simulink model "dynamical_model"  (R2023b)
settings: Solver=VariableStepAuto  StartTime=0.0  StopTime=10.0  RelTol=1e-3
values from neighbouring files (symbols this model uses):
  A = double(subs(A,[Lr lp Jr_ex mp Jp g Ke Kc Ra Br Bp],[Lr_ lp_ Jr_ex_ mp_ Jp_ g_ Ke_ Kc_ Ra_ Br_ Bp_]))    [linearized_mechanical_model.m]
  alpha_0 = 0    [DC_motor_and_Rod.m]    (also in linearized_mechanical_model.m)
  B = double(subs(B,[Lr lp Jr_ex mp Jp g Ke Kc Ra Br Bp],[Lr_ lp_ Jr_ex_ mp_ Jp_ g_ Ke_ Kc_ Ra_ Br_ Bp_]))    [linearized_mechanical_model.m]
  Bp_ = 1.25e-5    (= 1.25e-05)    [DC_motor_and_Rod.m]    (also in linearized_mechanical_model.m = 0)
  Br_ = 1.25e-5    (= 1.25e-05)    [DC_motor_and_Rod.m]    (also in linearized_mechanical_model.m = 0)
  C = [1,0,0,0 ... (first row only)    [linearized_mechanical_model.m]
  D = [0 ... (first row only)    [linearized_mechanical_model.m]
  g_ = 9.81    [DC_motor_and_Rod.m]    (also in linearized_mechanical_model.m)
  Jp_ = (1/12)*mp_*(3*rp^2 + Lp^2)    (= 3.3718538025e-05)    [DC_motor_and_Rod.m]    (also in linearized_mechanical_model.m = 2.44e-05)
  Jr_ex_ = 9.5e-5 + Jm    (= 9.96e-05)    [DC_motor_and_Rod.m]    (also in linearized_mechanical_model.m = 9.5e-05)
  Kc_ = 0.042    [DC_motor_and_Rod.m]    (also in linearized_mechanical_model.m)
  Ke_ = 0.042    [DC_motor_and_Rod.m]    (also in linearized_mechanical_model.m)
  lp_ = 0.95*Lp/2    (= 0.061275)    [DC_motor_and_Rod.m]    (also in linearized_mechanical_model.m = 0.0645)
  Lr_ = 0.09    [DC_motor_and_Rod.m]    (also in linearized_mechanical_model.m = 0.085)
  mp_ = 0.02421    [DC_motor_and_Rod.m]    (also in linearized_mechanical_model.m = 0.024)
  Ra_ = 8.4    [DC_motor_and_Rod.m]    (also in linearized_mechanical_model.m)
  theta_0 = 0    [DC_motor_and_Rod.m]    (also in linearized_mechanical_model.m)
  Va_0 = 0    [linearized_mechanical_model.m]
settings Model: Creator=renzo  LastModifiedBy=renzo

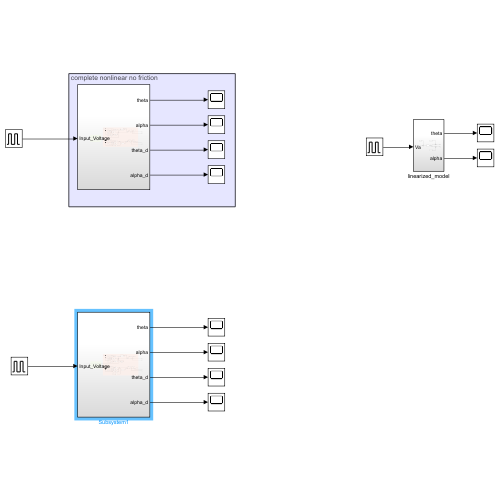
[thumbnail: Simulink's stored preview of the top-level diagram]
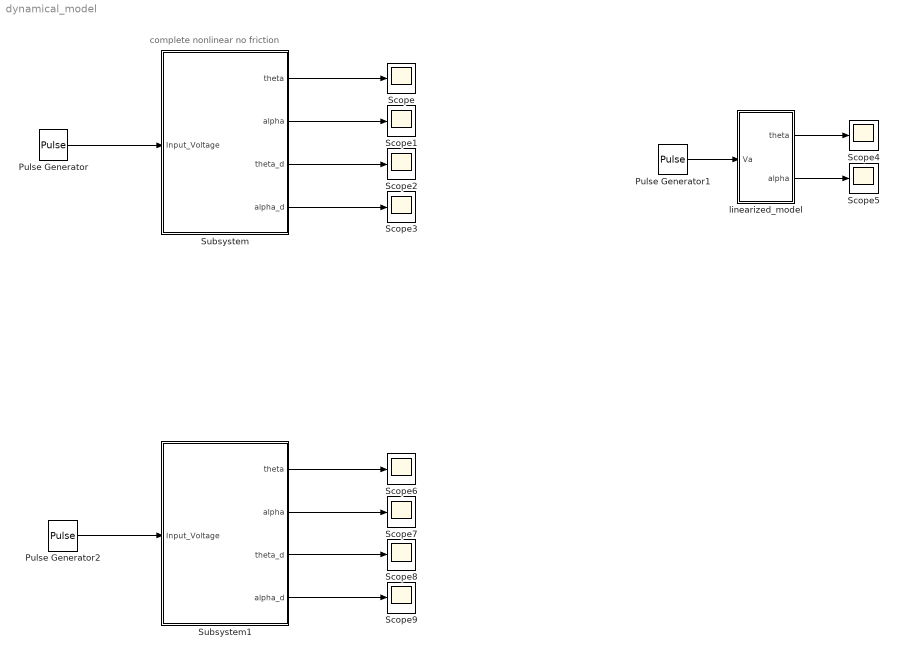
== system dynamical_model ==
  note: complete nonlinear no friction
  Pulse Generator : DiscretePulseGenerator  PulseType=Time based  Period=10
  Pulse Generator1 : DiscretePulseGenerator  PulseType=Time based  Period=10
  Pulse Generator2 : DiscretePulseGenerator  PulseType=Time based  Period=10
  Scope{,1..9} (10 alike) : Scope
  Subsystem : Subsystem
  Subsystem1 : Subsystem
  linearized_model : Subsystem
  wires:
  Pulse Generator/1 -> Subsystem/1(Input_Voltage)
  Subsystem/1(theta) -> Scope/1
  Subsystem/2(alpha) -> Scope1/1
  Subsystem/3(theta_d) -> Scope2/1
  Subsystem/4(alpha_d) -> Scope3/1
  Pulse Generator1/1 -> linearized_model/1(Va)
  linearized_model/1(theta) -> Scope4/1
  linearized_model/2(alpha) -> Scope5/1
  Subsystem1/4(alpha_d) -> Scope9/1
  Subsystem1/3(theta_d) -> Scope8/1
  Subsystem1/2(alpha) -> Scope7/1
  Subsystem1/1(theta) -> Scope6/1
  Pulse Generator2/1 -> Subsystem1/1(Input_Voltage)

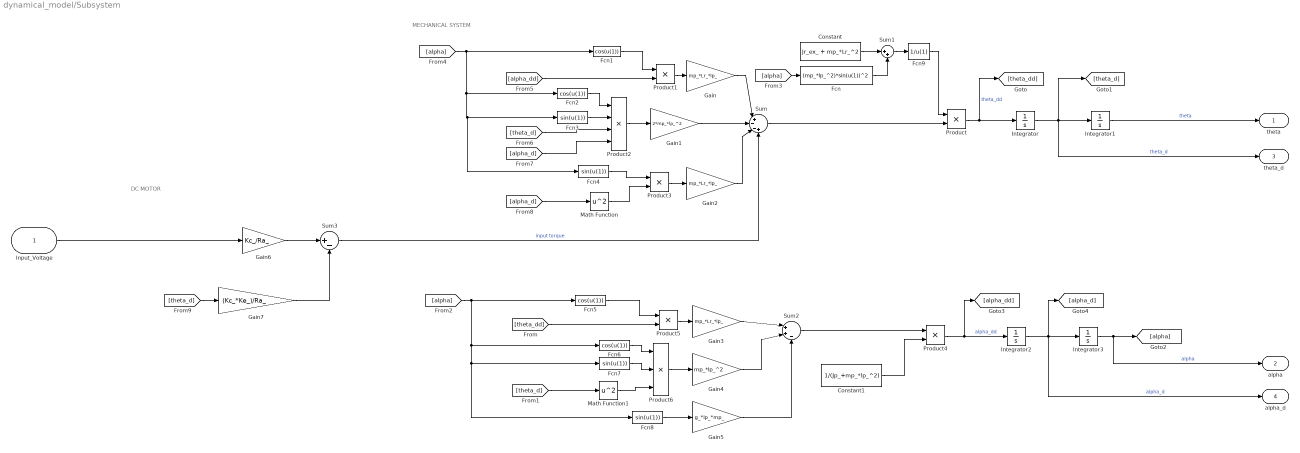
== system dynamical_model/Subsystem ==
  note: DC MOTOR
  note: MECHANICAL SYSTEM
  Input_Voltage : Inport
  Constant : Constant  Value=Jr_ex_ + mp_*Lr_^2
  Constant1 : Constant  Value=1/(Jp_+mp_*lp_^2)
  Fcn : Fcn  Expr=(mp_*lp_^2)*sin(u(1))^2
  Fcn{1..2,5..6} (4 alike) : Fcn  Expr=cos(u(1))
  Fcn{3..4,7..8} (4 alike) : Fcn  Expr=sin(u(1))
  Fcn9 : Fcn  Expr=1/u(1)
  Gain : Gain  Gain=mp_*Lr_*lp_
  Gain1 : Gain  Gain=2*mp_*lp_^2
  Gain2 : Gain  Gain=mp_*Lr_*lp_
  Gain3 : Gain  Gain=mp_*Lr_*lp_
  Gain4 : Gain  Gain=mp_*lp_^2
  Gain5 : Gain  Gain=g_*lp_*mp_
  Gain6 : Gain  Gain=Kc_/Ra_
  Gain7 : Gain  Gain=(Kc_*Ke_)/Ra_
  Integrator{,1..3} (4 alike) : Integrator
  Math Function : Math  Operator=square
  Math Function1 : Math  Operator=square
  Product{,1,3..5} (5 alike) : Product
  Product2 : Product  Inputs=4
  Product6 : Product  Inputs=3
  Sum : Sum  Inputs=|+--+
  Sum1 : Sum  Inputs=|++
  Sum2 : Sum  Inputs=|++-
  Sum3 : Sum  Inputs=|+-
  theta : Outport
  alpha : Outport  Port=2
  theta_d : Outport  Port=3
  alpha_d : Outport  Port=4
  wires:
  Integrator2/1 -> alpha_d/1, Integrator3/1, [alpha_d]  "alpha_d"
  Fcn6/1 -> Product6/1
  Product4/1 -> [alpha_dd], Integrator2/1  "alpha_dd"
  Fcn4/1 -> Product3/1
  Integrator/1 -> theta_d/1, [theta_d], Integrator1/1  "theta_d"
  Gain1/1 -> Sum/2
  Gain6/1 -> Sum3/1
  Fcn3/1 -> Product2/2
  Fcn1/1 -> Product1/1
  Integrator1/1 -> theta/1  "theta"
  Fcn8/1 -> Gain5/1
  Fcn7/1 -> Product6/2
  Gain5/1 -> Sum2/3
  Sum1/1 -> Fcn9/1
  Fcn/1 -> Sum1/2
  Product1/1 -> Gain/1
  Fcn9/1 -> Product/1
  Product3/1 -> Gain2/1
  Sum/1 -> Product/2
  [alpha_d] -> Math Function/1
  [theta_dd] -> Product5/2
  [theta_d] -> Gain7/1
  Product5/1 -> Gain3/1
  Integrator3/1 -> alpha/1, [alpha]  "alpha"
  Fcn5/1 -> Product5/1
  Product6/1 -> Gain4/1
  Sum2/1 -> Product4/1
  Math Function1/1 -> Product6/3
  Math Function/1 -> Product3/2
  Product/1 -> Integrator/1, [theta_dd]  "theta_dd"
  Gain4/1 -> Sum2/2
  Input_Voltage/1 -> Gain6/1
  Constant/1 -> Sum1/1
  [alpha] -> Fcn8/1, Fcn7/1, Fcn6/1, Fcn5/1
  Constant1/1 -> Product4/2
  Product2/1 -> Gain1/1
  [alpha] -> Fcn4/1, Fcn3/1, Fcn2/1, Fcn1/1
  [alpha_d] -> Product2/4
  [alpha_dd] -> Product1/2
  [alpha] -> Fcn/1
  Fcn2/1 -> Product2/1
  Sum3/1 -> Sum/4  "input torque"
  Gain2/1 -> Sum/3
  Gain/1 -> Sum/1
  Gain3/1 -> Sum2/1
  [theta_d] -> Math Function1/1
  Gain7/1 -> Sum3/2
  [theta_d] -> Product2/3

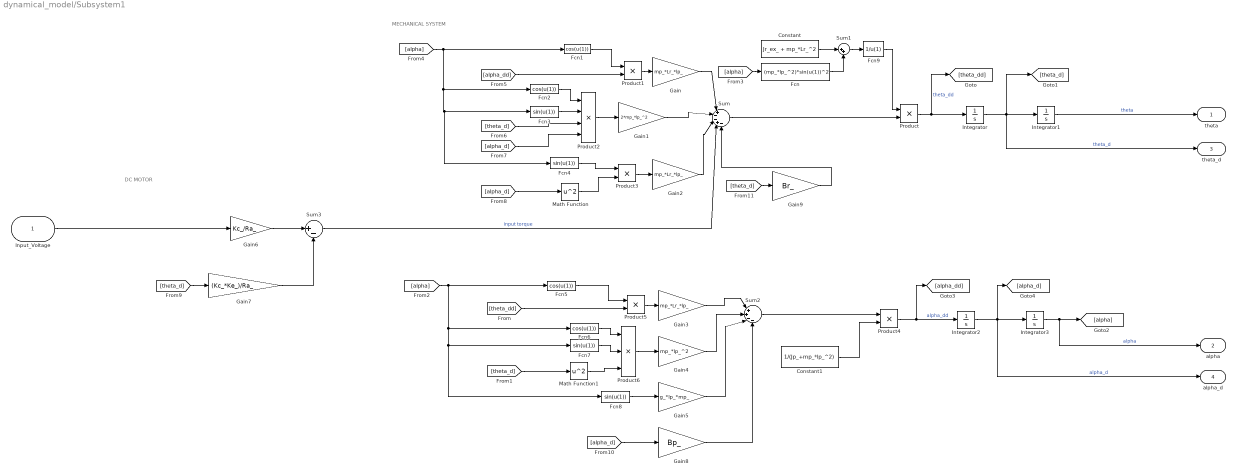
== system dynamical_model/Subsystem1 ==
  note: MECHANICAL SYSTEM
  note: DC MOTOR
  Input_Voltage : Inport
  Constant : Constant  Value=Jr_ex_ + mp_*Lr_^2
  Constant1 : Constant  Value=1/(Jp_+mp_*lp_^2)
  Fcn : Fcn  Expr=(mp_*lp_^2)*sin(u(1))^2
  Fcn{1..2,5..6} (4 alike) : Fcn  Expr=cos(u(1))
  Fcn{3..4,7..8} (4 alike) : Fcn  Expr=sin(u(1))
  Fcn9 : Fcn  Expr=1/u(1)
  Gain : Gain  Gain=mp_*Lr_*lp_
  Gain1 : Gain  Gain=2*mp_*lp_^2
  Gain2 : Gain  Gain=mp_*Lr_*lp_
  Gain3 : Gain  Gain=mp_*Lr_*lp_
  Gain4 : Gain  Gain=mp_*lp_^2
  Gain5 : Gain  Gain=g_*lp_*mp_
  Gain6 : Gain  Gain=Kc_/Ra_
  Gain7 : Gain  Gain=(Kc_*Ke_)/Ra_
  Gain8 : Gain  Gain=Bp_
  Gain9 : Gain  Gain=Br_
  Integrator{,1..3} (4 alike) : Integrator
  Math Function : Math  Operator=square
  Math Function1 : Math  Operator=square
  Product{,1,3..5} (5 alike) : Product
  Product2 : Product  Inputs=4
  Product6 : Product  Inputs=3
  Sum : Sum  Inputs=|+--+-
  Sum1 : Sum  Inputs=|++
  Sum2 : Sum  Inputs=|++--
  Sum3 : Sum  Inputs=|+-
  theta : Outport
  alpha : Outport  Port=2
  theta_d : Outport  Port=3
  alpha_d : Outport  Port=4
  wires:
  [theta_d] -> Product2/3
  Gain7/1 -> Sum3/2
  [theta_d] -> Math Function1/1
  Gain3/1 -> Sum2/1
  Gain/1 -> Sum/1
  Gain2/1 -> Sum/3
  Sum3/1 -> Sum/4  "input torque"
  Fcn2/1 -> Product2/1
  [alpha] -> Fcn/1
  [alpha_dd] -> Product1/2
  [alpha_d] -> Product2/4
  [alpha] -> Fcn1/1, Fcn2/1, Fcn3/1, Fcn4/1
  Product2/1 -> Gain1/1
  Constant1/1 -> Product4/2
  [alpha] -> Fcn5/1, Fcn6/1, Fcn7/1, Fcn8/1
  Constant/1 -> Sum1/1
  Input_Voltage/1 -> Gain6/1
  Gain4/1 -> Sum2/2
  Product/1 -> [theta_dd], Integrator/1  "theta_dd"
  Math Function/1 -> Product3/2
  Math Function1/1 -> Product6/3
  Sum2/1 -> Product4/1
  Product6/1 -> Gain4/1
  Fcn5/1 -> Product5/1
  Integrator3/1 -> [alpha], alpha/1  "alpha"
  Product5/1 -> Gain3/1
  [theta_d] -> Gain7/1
  [theta_dd] -> Product5/2
  [alpha_d] -> Math Function/1
  Sum/1 -> Product/2
  Product3/1 -> Gain2/1
  Fcn9/1 -> Product/1
  Product1/1 -> Gain/1
  Fcn/1 -> Sum1/2
  Sum1/1 -> Fcn9/1
  Gain5/1 -> Sum2/3
  Fcn7/1 -> Product6/2
  Fcn8/1 -> Gain5/1
  Integrator1/1 -> theta/1  "theta"
  Fcn1/1 -> Product1/1
  Fcn3/1 -> Product2/2
  Gain6/1 -> Sum3/1
  Gain1/1 -> Sum/2
  Integrator/1 -> Integrator1/1, [theta_d], theta_d/1  "theta_d"
  Fcn4/1 -> Product3/1
  Product4/1 -> Integrator2/1, [alpha_dd]  "alpha_dd"
  Fcn6/1 -> Product6/1
  Integrator2/1 -> [alpha_d], Integrator3/1, alpha_d/1  "alpha_d"
  [alpha_d] -> Gain8/1
  Gain8/1 -> Sum2/4
  [theta_d] -> Gain9/1
  Gain9/1 -> Sum/5

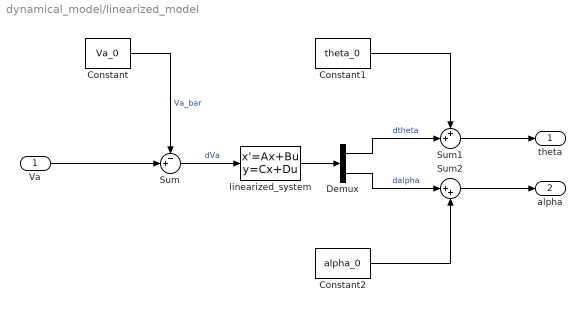
== system dynamical_model/linearized_model ==
  Va : Inport
  Constant : Constant  Value=Va_0
  Constant1 : Constant  Value=theta_0
  Constant2 : Constant  Value=alpha_0
  Demux : Demux  Outputs=2
  Sum : Sum  Inputs=-+|
  Sum1 : Sum  Inputs=++|
  Sum2 : Sum  Inputs=|++
  linearized_system : StateSpace  A=A  B=B  C=C  D=D  InitialCondition=0
  theta : Outport
  alpha : Outport  Port=2
  wires:
  Va/1 -> Sum/2
  Demux/1 -> Sum1/2  "dtheta"
  linearized_system/1 -> Demux/1
  Constant/1 -> Sum/1  "Va_bar"
  Sum/1 -> linearized_system/1  "dVa"
  Constant1/1 -> Sum1/1
  Constant2/1 -> Sum2/2
  Sum2/1 -> alpha/1
  Demux/2 -> Sum2/1  "dalpha"
  Sum1/1 -> theta/1
